simulink model "Matrix12"  (R2021a)
settings: Solver=VariableStepAuto  StartTime=0.0  StopTime=1  RelTol=1e-3
undefined symbols (not defined in the file): DiscIntNeverNeededParam
libraries: spsDiodeLib x18, spsIGBTLib x18, simulink x6, spsIGBTDiodeLib x6, spsSeriesRLCBranchLib x4, spsThreePhaseVIMeasurementLib x3, spsSaturableTransformerLib x3, spsabctoAlphaBetaZeroLib x2, spsAlphaBetaZerotoabcLib x1, pid_lib x1, spsSecondOrderFilterLib x1, spsThreePhaseSeriesRLCBranchLib x1
(part 2 of 2)

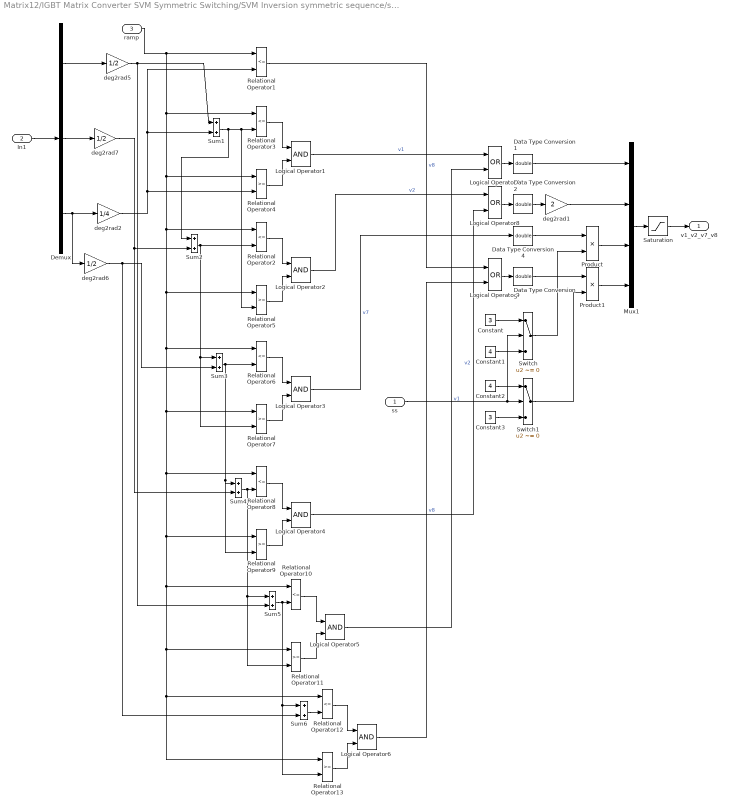
== system Matrix12/IGBT Matrix Converter SVM Symmetric Switching/SVM Inversion symmetric sequence/symmetric sequence ==
  ss : Inport
  In1 : Inport  Port=2
  ramp : Inport  Port=3
  Constant : Constant  Value=3
  Constant1 : Constant  Value=4
  Constant2 : Constant  Value=4
  Constant3 : Constant  Value=3
  Data Type Conversion{1..2,4..5} (4 alike) : DataTypeConversion  OutDataTypeStr=double
  Demux : Demux  Outputs=3
  Logical Operator{1..6} (6 alike) : Logic  AllPortsSameDT=off  OutDataTypeStr=boolean
  Logical Operator7 : Logic  Operator=OR  AllPortsSameDT=off  OutDataTypeStr=boolean
  Logical Operator8 : Logic  Operator=OR  AllPortsSameDT=off  OutDataTypeStr=boolean
  Logical Operator9 : Logic  Operator=OR  AllPortsSameDT=off  OutDataTypeStr=boolean
  Mux1 : Mux
  Product : Product  RndMeth=Zero
  Product1 : Product  RndMeth=Zero
  Relational Operator{1..3,6,8,10,12} (7 alike) : RelationalOperator  Operator=<=  RndMeth=Nearest  InputSameDT=on
  Relational Operator{4..5,7,9,11,13} (6 alike) : RelationalOperator  RndMeth=Nearest  InputSameDT=on
  Saturation : Saturate  UpperLimit=4  LowerLimit=1
  Sum{1..6} (6 alike) : Sum
  Switch : Switch  Criteria=u2 ~= 0
  Switch1 : Switch  Criteria=u2 ~= 0
  deg2rad1 : Gain  Gain=2
  deg2rad2 : Gain  Gain=1/4
  deg2rad5 : Gain  Gain=1/2
  deg2rad6 : Gain  Gain=1/2
  deg2rad7 : Gain  Gain=1/2
  v1_v2_v7_v8 : Outport  VectorParamsAs1DForOutWhenUnconnected=off
  wires:
  ss/1 -> Switch/2, Switch1/2
  Switch1/1 -> Product1/2
  Switch/1 -> Product/2
  Constant2/1 -> Switch1/1
  Constant3/1 -> Switch1/3
  Constant/1 -> Switch/1
  Constant1/1 -> Switch/3
  Product1/1 -> Mux1/4
  Product/1 -> Mux1/3
  Data Type Conversion5/1 -> Product1/1
  Data Type Conversion4/1 -> Product/1
  Data Type Conversion2/1 -> deg2rad1/1
  Data Type Conversion1/1 -> Mux1/1
  Logical Operator7/1 -> Data Type Conversion1/1
  Relational Operator1/1 -> Logical Operator9/1  "v8"
  Logical Operator1/1 -> Logical Operator7/1  "v1"
  Logical Operator6/1 -> Logical Operator9/2  "v8"
  Sum6/1 -> Relational Operator12/2
  Relational Operator13/1 -> Logical Operator6/2
  Relational Operator12/1 -> Logical Operator6/1
  Logical Operator5/1 -> Logical Operator7/2  "v1"
  Sum5/1 -> Relational Operator13/2, Sum6/1, Relational Operator10/2
  Relational Operator11/1 -> Logical Operator5/2
  Relational Operator10/1 -> Logical Operator5/1
  Logical Operator4/1 -> Logical Operator8/2  "v2"
  deg2rad7/1 -> Sum2/2, Sum4/2
  Demux/2 -> deg2rad7/1
  Sum4/1 -> Sum5/1, Relational Operator11/2, Relational Operator8/2
  Relational Operator9/1 -> Logical Operator4/2
  Relational Operator8/1 -> Logical Operator4/1
  deg2rad6/1 -> Sum6/2, Sum3/2
  Sum3/1 -> Relational Operator9/2, Sum4/1, Relational Operator6/2
  Logical Operator3/1 -> Data Type Conversion4/1  "v7"
  Relational Operator7/1 -> Logical Operator3/2
  Relational Operator6/1 -> Logical Operator3/1
  Logical Operator2/1 -> Logical Operator8/1  "v2"
  Sum2/1 -> Relational Operator7/2, Sum3/1, Relational Operator2/2
  Relational Operator5/1 -> Logical Operator2/2
  Relational Operator2/1 -> Logical Operator2/1
  deg2rad5/1 -> Sum5/2, Sum1/1
  Demux/1 -> deg2rad5/1
  deg2rad2/1 -> Sum1/2, Relational Operator1/2, Relational Operator4/2
  Sum1/1 -> Sum2/1, Relational Operator5/2, Relational Operator3/2
  Relational Operator4/1 -> Logical Operator1/2
  Relational Operator3/1 -> Logical Operator1/1
  Saturation/1 -> v1_v2_v7_v8/1
  Logical Operator9/1 -> Data Type Conversion5/1
  Logical Operator8/1 -> Data Type Conversion2/1
  deg2rad1/1 -> Mux1/2
  In1/1 -> Demux/1
  ramp/1 -> Relational Operator1/1, Relational Operator13/1, Relational Operator12/1, Relational Operator11/1, Relational Operator10/1, Relational Operator9/1, Relational Operator8/1, Relational Operator7/1, Relational Operator6/1, Relational Operator5/1, Relational Operator2/1, Relational Operator4/1, Relational Operator3/1
  Mux1/1 -> Saturation/1
  Demux/3 -> deg2rad6/1, deg2rad2/1

== system Matrix12/IGBT Matrix Converter SVM Symmetric Switching/SVM Rectification symmetric sequence/Calculate duty-cycles ==
  deg_mag : Inport
  Trigger : TriggerPort  VariantControl=Variant
  Constant : Constant  Value=pi/3
  Constant1 : Constant
  Demux : Demux  Outputs=2
  Mux : Mux  Inputs=2
  Mux1 : Mux  Inputs=2
  Product : Product  Inputs=**  RndMeth=Zero
  Sum : Sum  Inputs=+-
  Sum of Elements : Sum  Inputs=+
  Sum1 : Sum  Inputs=-+
  Sum2 : Sum  Inputs=-+
  Trigonometric Function : Trigonometry  Operator=cos
  Trigonometric Function1 : Trigonometry
  deg2rad : Gain  Gain=pi/180
  deg2rad1 : Gain  Gain=0.5/0.866
  d1_d2_d0 : Outport  VectorParamsAs1DForOutWhenUnconnected=off
  wires:
  Sum of Elements/1 -> Sum2/1
  Constant1/1 -> Sum2/2
  Sum2/1 -> Mux1/2  "d0"
  Mux1/1 -> d1_d2_d0/1
  Product/1 -> Sum of Elements/1, Mux1/1  "d1 d2"
  Constant/1 -> Sum1/2
  Mux/1 -> Trigonometric Function1/1, Trigonometric Function/1
  Sum1/1 -> Mux/2
  deg2rad/1 -> Sum1/1, Mux/1  "theta"
  Sum/1 -> Product/1
  deg2rad1/1 -> Sum/2
  Trigonometric Function1/1 -> deg2rad1/1
  Trigonometric Function/1 -> Sum/1
  Demux/2 -> Product/2  "mag"
  Demux/1 -> deg2rad/1
  deg_mag/1 -> Demux/1

== system Matrix12/IGBT Matrix Converter SVM Symmetric Switching/SVM Rectification symmetric sequence/Triggered Subsystem ==
  In1 : Inport
  Trigger : TriggerPort  VariantControl=Variant
  Out1 : Outport  VectorParamsAs1DForOutWhenUnconnected=off
  wires:
  In1/1 -> Out1/1

== system Matrix12/IGBT Matrix Converter SVM Symmetric Switching/SVM Rectification symmetric sequence/abc 2 alpha-beta ==
  Vabc : Inport
  Demux : Demux  Outputs=3
      settings: DisplayOption=none
  Gain : Gain  Gain=1/2  SaturateOnIntegerOverflow=on  OutDataTypeStr=Inherit: Same as input  ParamDataTypeStr=Inherit: Same as input
  Gain1 : Gain  Gain=1/2  SaturateOnIntegerOverflow=on  OutDataTypeStr=Inherit: Same as input  ParamDataTypeStr=Inherit: Same as input
  Gain2 : Gain  Gain=sqrt(2/3)  SaturateOnIntegerOverflow=on  OutDataTypeStr=Inherit: Same as input  ParamDataTypeStr=Inherit: Same as input
  Gain3 : Gain  Gain=sqrt(3)/2  SaturateOnIntegerOverflow=on  OutDataTypeStr=Inherit: Same as input  ParamDataTypeStr=Inherit: Same as input
  Gain4 : Gain  Gain=sqrt(3)/2  SaturateOnIntegerOverflow=on  OutDataTypeStr=Inherit: Same as input  ParamDataTypeStr=Inherit: Same as input
  Gain5 : Gain  Gain=sqrt(2/3)  SaturateOnIntegerOverflow=on  OutDataTypeStr=Inherit: Same as input  ParamDataTypeStr=Inherit: Same as input
  Sum : Sum  Inputs=+--  InputSameDT=on  SaturateOnIntegerOverflow=on  OutDataTypeStr=Inherit: Same as first input
  Sum1 : Sum  Inputs=+-  InputSameDT=on  SaturateOnIntegerOverflow=on  OutDataTypeStr=Inherit: Same as first input
  Valpha : Outport  VectorParamsAs1DForOutWhenUnconnected=off
  Vbeta : Outport  Port=2  VectorParamsAs1DForOutWhenUnconnected=off
  wires:
  Gain5/1 -> Vbeta/1
  Gain2/1 -> Valpha/1
  Vabc/1 -> Demux/1
  Gain3/1 -> Sum1/1
  Gain4/1 -> Sum1/2
  Sum1/1 -> Gain5/1
  Sum/1 -> Gain2/1
  Gain1/1 -> Sum/3
  Gain/1 -> Sum/2
  Demux/1 -> Sum/1
  Demux/2 -> Gain/1, Gain3/1
  Demux/3 -> Gain1/1, Gain4/1

== system Matrix12/IGBT Matrix Converter SVM Symmetric Switching/SVM Rectification symmetric sequence/alpha-beta 2 deg-mag ==
  Valpha : Inport
  Vbeta : Inport  Port=2
  Constant1 : Constant  Value=180
  Constant2 : Constant  Value=-360
  Constant20 : Constant  Value=30
  Math Function : Math  Operator=square  SignedPower=on  SaturateOnIntegerOverflow=on
  Math Function1 : Math  Operator=sqrt  SignedPower=on  SaturateOnIntegerOverflow=on
  Mux1 : Mux  Inputs=2
  Relational Operator2 : RelationalOperator  Operator=>  RndMeth=Nearest  InputSameDT=on
  Sum of Elements : Sum  Inputs=+
  Sum1 : Sum  Inputs=|++
  Sum2 : Sum  Inputs=|++
  Switch : Switch  Criteria=u2 ~= 0
  Trigonometric Function : Trigonometry  Operator=atan2
  rad2deg : Gain  Gain=180/pi  SaturateOnIntegerOverflow=on  OutDataTypeStr=Inherit: Same as input  ParamDataTypeStr=Inherit: Same as input
  Vdeg : Outport  VectorParamsAs1DForOutWhenUnconnected=off
  Vmag : Outport  Port=2  VectorParamsAs1DForOutWhenUnconnected=off
  wires:
  Trigonometric Function/1 -> rad2deg/1
  Valpha/1 -> Trigonometric Function/2, Mux1/1
  Mux1/1 -> Math Function/1
  Math Function/1 -> Sum of Elements/1
  Sum of Elements/1 -> Math Function1/1
  Vbeta/1 -> Trigonometric Function/1, Mux1/2
  Math Function1/1 -> Vmag/1
  rad2deg/1 -> Sum1/1
  Constant20/1 -> Sum1/2
  Sum1/1 -> Relational Operator2/1, Switch/3, Sum2/1
  Relational Operator2/1 -> Switch/2
  Switch/1 -> Vdeg/1
  Constant1/1 -> Relational Operator2/2
  Sum2/1 -> Switch/1
  Constant2/1 -> Sum2/2

== system Matrix12/IGBT Matrix Converter SVM Symmetric Switching/SVM Rectification symmetric sequence/choose zero-vector ==
  sector : Inport
  Compare To Constant : simulink/Logic and Bit Operations/Compare To Constant  relop===  const=1  OutDataTypeStr=uint8  ZeroCross=off
  Compare To Constant1 : simulink/Logic and Bit Operations/Compare To Constant  relop===  const=4  OutDataTypeStr=uint8  ZeroCross=off
  Compare To Constant2 : simulink/Logic and Bit Operations/Compare To Constant  relop===  const=2  OutDataTypeStr=uint8  ZeroCross=off
  Compare To Constant3 : simulink/Logic and Bit Operations/Compare To Constant  relop===  const=5  OutDataTypeStr=uint8  ZeroCross=off
  Compare To Constant4 : simulink/Logic and Bit Operations/Compare To Constant  relop===  const=3  OutDataTypeStr=uint8  ZeroCross=off
  Compare To Constant5 : simulink/Logic and Bit Operations/Compare To Constant  relop===  const=6  OutDataTypeStr=uint8  ZeroCross=off
  Data Type Conversion1 : DataTypeConversion  OutDataTypeStr=double
  Data Type Conversion2 : DataTypeConversion  OutDataTypeStr=double
  Data Type Conversion3 : DataTypeConversion  OutDataTypeStr=double
  Logical Operator1 : Logic  Operator=OR  AllPortsSameDT=off  OutDataTypeStr=boolean
  Logical Operator2 : Logic  Operator=OR  AllPortsSameDT=off  OutDataTypeStr=boolean
  Logical Operator8 : Logic  Operator=OR  AllPortsSameDT=off  OutDataTypeStr=boolean
  MinMax1 : MinMax  Function=max
  Mux1 : Mux  Inputs=3
  Saturation1 : Saturate  UpperLimit=3  LowerLimit=1
  deg2rad2 : Gain  Gain=2
  deg2rad4 : Gain  Gain=3
  zv : Outport  VectorParamsAs1DForOutWhenUnconnected=off
  wires:
  Compare To Constant/1 -> Logical Operator8/1
  Compare To Constant1/1 -> Logical Operator8/2
  Compare To Constant2/1 -> Logical Operator1/1
  Compare To Constant3/1 -> Logical Operator1/2
  Compare To Constant4/1 -> Logical Operator2/1
  Compare To Constant5/1 -> Logical Operator2/2
  Logical Operator8/1 -> Data Type Conversion1/1
  Logical Operator1/1 -> Data Type Conversion2/1
  Logical Operator2/1 -> Data Type Conversion3/1
  Data Type Conversion1/1 -> Mux1/1
  Data Type Conversion2/1 -> deg2rad2/1
  Data Type Conversion3/1 -> deg2rad4/1
  Mux1/1 -> Saturation1/1
  deg2rad4/1 -> Mux1/3
  deg2rad2/1 -> Mux1/2
  Saturation1/1 -> MinMax1/1
  MinMax1/1 -> zv/1
  sector/1 -> Compare To Constant/1, Compare To Constant1/1, Compare To Constant2/1, Compare To Constant3/1, Compare To Constant4/1, Compare To Constant5/1

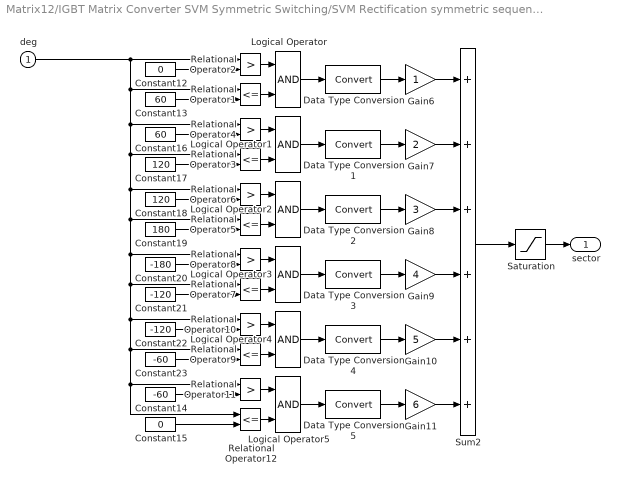
== system Matrix12/IGBT Matrix Converter SVM Symmetric Switching/SVM Rectification symmetric sequence/sector ==
  deg : Inport
  Constant12 : Constant  Value=0
  Constant13 : Constant  Value=60
  Constant14 : Constant  Value=-60
  Constant15 : Constant  Value=0
  Constant16 : Constant  Value=60
  Constant17 : Constant  Value=120
  Constant18 : Constant  Value=120
  Constant19 : Constant  Value=180
  Constant20 : Constant  Value=-180
  Constant21 : Constant  Value=-120
  Constant22 : Constant  Value=-120
  Constant23 : Constant  Value=-60
  Data Type Conversion{,1..5} (6 alike) : DataTypeConversion  SaturateOnIntegerOverflow=on  RndMeth=Zero
  Gain10 : Gain  Gain=5  SaturateOnIntegerOverflow=on  OutDataTypeStr=Inherit: Same as input  ParamDataTypeStr=Inherit: Same as input
  Gain11 : Gain  Gain=6  SaturateOnIntegerOverflow=on  OutDataTypeStr=Inherit: Same as input  ParamDataTypeStr=Inherit: Same as input
  Gain6 : Gain  SaturateOnIntegerOverflow=on  OutDataTypeStr=Inherit: Same as input  ParamDataTypeStr=Inherit: Same as input
  Gain7 : Gain  Gain=2  SaturateOnIntegerOverflow=on  OutDataTypeStr=Inherit: Same as input  ParamDataTypeStr=Inherit: Same as input
  Gain8 : Gain  Gain=3  SaturateOnIntegerOverflow=on  OutDataTypeStr=Inherit: Same as input  ParamDataTypeStr=Inherit: Same as input
  Gain9 : Gain  Gain=4  SaturateOnIntegerOverflow=on  OutDataTypeStr=Inherit: Same as input  ParamDataTypeStr=Inherit: Same as input
  Logical Operator{,1..5} (6 alike) : Logic
  Relational Operator{1,3,5,7,9,12} (6 alike) : RelationalOperator  Operator=<=  RndMeth=Nearest  InputSameDT=on
  Relational Operator{2,4,6,8,10..11} (6 alike) : RelationalOperator  Operator=>  RndMeth=Nearest  InputSameDT=on
  Saturation : Saturate  UpperLimit=6  LowerLimit=1
  Sum2 : Sum  Inputs=++++++  InputSameDT=on  SaturateOnIntegerOverflow=on  OutDataTypeStr=Inherit: Same as first input
  sector : Outport  VectorParamsAs1DForOutWhenUnconnected=off
  wires:
  deg/1 -> Relational Operator2/1, Relational Operator1/1, Relational Operator4/1, Relational Operator3/1, Relational Operator6/1, Relational Operator5/1, Relational Operator8/1, Relational Operator7/1, Relational Operator10/1, Relational Operator9/1, Relational Operator11/1, Relational Operator12/1
  Saturation/1 -> sector/1
  Data Type Conversion5/1 -> Gain11/1
  Data Type Conversion4/1 -> Gain10/1
  Data Type Conversion3/1 -> Gain9/1
  Data Type Conversion2/1 -> Gain8/1
  Data Type Conversion1/1 -> Gain7/1
  Data Type Conversion/1 -> Gain6/1
  Relational Operator2/1 -> Logical Operator/1
  Relational Operator1/1 -> Logical Operator/2
  Logical Operator/1 -> Data Type Conversion/1
  Constant12/1 -> Relational Operator2/2
  Constant13/1 -> Relational Operator1/2
  Relational Operator4/1 -> Logical Operator1/1
  Relational Operator3/1 -> Logical Operator1/2
  Logical Operator1/1 -> Data Type Conversion1/1
  Constant16/1 -> Relational Operator4/2
  Constant17/1 -> Relational Operator3/2
  Relational Operator6/1 -> Logical Operator2/1
  Relational Operator5/1 -> Logical Operator2/2
  Logical Operator2/1 -> Data Type Conversion2/1
  Constant18/1 -> Relational Operator6/2
  Constant19/1 -> Relational Operator5/2
  Relational Operator8/1 -> Logical Operator3/1
  Relational Operator7/1 -> Logical Operator3/2
  Logical Operator3/1 -> Data Type Conversion3/1
  Constant20/1 -> Relational Operator8/2
  Constant21/1 -> Relational Operator7/2
  Relational Operator10/1 -> Logical Operator4/1
  Relational Operator9/1 -> Logical Operator4/2
  Logical Operator4/1 -> Data Type Conversion4/1
  Constant22/1 -> Relational Operator10/2
  Constant23/1 -> Relational Operator9/2
  Relational Operator11/1 -> Logical Operator5/1
  Relational Operator12/1 -> Logical Operator5/2
  Logical Operator5/1 -> Data Type Conversion5/1
  Constant14/1 -> Relational Operator11/2
  Constant15/1 -> Relational Operator12/2
  Gain6/1 -> Sum2/1
  Gain7/1 -> Sum2/2
  Gain8/1 -> Sum2/3
  Gain9/1 -> Sum2/4
  Gain10/1 -> Sum2/5
  Gain11/1 -> Sum2/6
  Sum2/1 -> Saturation/1

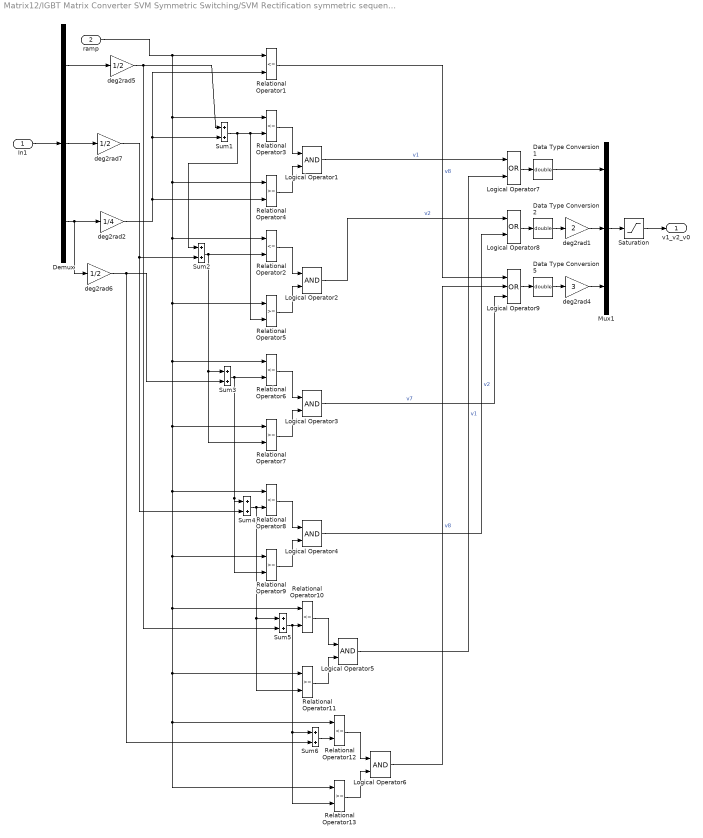
== system Matrix12/IGBT Matrix Converter SVM Symmetric Switching/SVM Rectification symmetric sequence/symmetric sequence ==
  In1 : Inport
  ramp : Inport  Port=2
  Data Type Conversion1 : DataTypeConversion  OutDataTypeStr=double
  Data Type Conversion2 : DataTypeConversion  OutDataTypeStr=double
  Data Type Conversion5 : DataTypeConversion  OutDataTypeStr=double
  Demux : Demux  Outputs=3
  Logical Operator{1..6} (6 alike) : Logic  AllPortsSameDT=off  OutDataTypeStr=boolean
  Logical Operator7 : Logic  Operator=OR  AllPortsSameDT=off  OutDataTypeStr=boolean
  Logical Operator8 : Logic  Operator=OR  AllPortsSameDT=off  OutDataTypeStr=boolean
  Logical Operator9 : Logic  Operator=OR  Inputs=3  AllPortsSameDT=off  OutDataTypeStr=boolean
  Mux1 : Mux  Inputs=3
  Relational Operator{1..3,6,8,10,12} (7 alike) : RelationalOperator  Operator=<=  RndMeth=Nearest  InputSameDT=on
  Relational Operator{4..5,7,9,11,13} (6 alike) : RelationalOperator  RndMeth=Nearest  InputSameDT=on
  Saturation : Saturate  UpperLimit=3  LowerLimit=1
  Sum{1..6} (6 alike) : Sum
  deg2rad1 : Gain  Gain=2
  deg2rad2 : Gain  Gain=1/4
  deg2rad4 : Gain  Gain=3
  deg2rad5 : Gain  Gain=1/2
  deg2rad6 : Gain  Gain=1/2
  deg2rad7 : Gain  Gain=1/2
  v1_v2_v0 : Outport  VectorParamsAs1DForOutWhenUnconnected=off
  wires:
  Demux/3 -> deg2rad2/1, deg2rad6/1
  Mux1/1 -> Saturation/1
  ramp/1 -> Relational Operator3/1, Relational Operator4/1, Relational Operator2/1, Relational Operator5/1, Relational Operator6/1, Relational Operator7/1, Relational Operator8/1, Relational Operator9/1, Relational Operator10/1, Relational Operator11/1, Relational Operator12/1, Relational Operator13/1, Relational Operator1/1
  In1/1 -> Demux/1
  deg2rad1/1 -> Mux1/2
  deg2rad4/1 -> Mux1/3
  Logical Operator8/1 -> Data Type Conversion2/1
  Logical Operator9/1 -> Data Type Conversion5/1
  Saturation/1 -> v1_v2_v0/1
  Relational Operator3/1 -> Logical Operator1/1
  Relational Operator4/1 -> Logical Operator1/2
  Sum1/1 -> Relational Operator3/2, Relational Operator5/2, Sum2/1
  deg2rad2/1 -> Relational Operator4/2, Relational Operator1/2, Sum1/2
  Demux/1 -> deg2rad5/1
  deg2rad5/1 -> Sum1/1, Sum5/2
  Relational Operator2/1 -> Logical Operator2/1
  Relational Operator5/1 -> Logical Operator2/2
  Sum2/1 -> Relational Operator2/2, Sum3/1, Relational Operator7/2
  Logical Operator2/1 -> Logical Operator8/1  "v2"
  Relational Operator6/1 -> Logical Operator3/1
  Relational Operator7/1 -> Logical Operator3/2
  Sum3/1 -> Relational Operator6/2, Sum4/1, Relational Operator9/2
  deg2rad6/1 -> Sum3/2, Sum6/2
  Relational Operator8/1 -> Logical Operator4/1
  Relational Operator9/1 -> Logical Operator4/2
  Sum4/1 -> Relational Operator8/2, Relational Operator11/2, Sum5/1
  Demux/2 -> deg2rad7/1
  deg2rad7/1 -> Sum4/2, Sum2/2
  Logical Operator4/1 -> Logical Operator8/2  "v2"
  Relational Operator10/1 -> Logical Operator5/1
  Relational Operator11/1 -> Logical Operator5/2
  Sum5/1 -> Relational Operator10/2, Sum6/1, Relational Operator13/2
  Logical Operator5/1 -> Logical Operator7/2  "v1"
  Relational Operator12/1 -> Logical Operator6/1
  Relational Operator13/1 -> Logical Operator6/2
  Sum6/1 -> Relational Operator12/2
  Logical Operator6/1 -> Logical Operator9/2  "v8"
  Logical Operator1/1 -> Logical Operator7/1  "v1"
  Relational Operator1/1 -> Logical Operator9/1  "v8"
  Logical Operator7/1 -> Data Type Conversion1/1
  Data Type Conversion1/1 -> Mux1/1
  Data Type Conversion2/1 -> deg2rad1/1
  Data Type Conversion5/1 -> deg2rad4/1
  Logical Operator3/1 -> Logical Operator9/3  "v7"

== system Matrix12/IGBT Matrix Converter SVM Symmetric Switching/matrix converter switching/Subsystem1 ==
  In1 : Inport
  In2 : Inport  Port=2
  In3 : Inport  Port=3
  In4 : Inport  Port=4
  Data Type Conversion : DataTypeConversion  OutDataTypeStr=double
  Logical Operator : Logic  AllPortsSameDT=off  OutDataTypeStr=boolean
  Logical Operator1 : Logic  AllPortsSameDT=off  OutDataTypeStr=boolean
  Logical Operator2 : Logic  Operator=OR  AllPortsSameDT=off  OutDataTypeStr=boolean
  Out1 : Outport  VectorParamsAs1DForOutWhenUnconnected=off
  wires:
  In4/1 -> Logical Operator1/2
  In3/1 -> Logical Operator1/1
  Logical Operator2/1 -> Data Type Conversion/1
  In2/1 -> Logical Operator/2
  In1/1 -> Logical Operator/1
  Logical Operator1/1 -> Logical Operator2/2
  Logical Operator/1 -> Logical Operator2/1
  Data Type Conversion/1 -> Out1/1

== system Matrix12/IGBT Matrix Converter SVM Symmetric Switching/matrix converter switching/Subsystem2 ==
  In1 : Inport
  In2 : Inport  Port=2
  In3 : Inport  Port=3
  In4 : Inport  Port=4
  Data Type Conversion : DataTypeConversion  OutDataTypeStr=double
  Logical Operator : Logic  AllPortsSameDT=off  OutDataTypeStr=boolean
  Logical Operator1 : Logic  AllPortsSameDT=off  OutDataTypeStr=boolean
  Logical Operator2 : Logic  Operator=OR  AllPortsSameDT=off  OutDataTypeStr=boolean
  Out1 : Outport  VectorParamsAs1DForOutWhenUnconnected=off
  wires:
  In4/1 -> Logical Operator1/2
  In3/1 -> Logical Operator1/1
  Logical Operator2/1 -> Data Type Conversion/1
  In2/1 -> Logical Operator/2
  In1/1 -> Logical Operator/1
  Logical Operator1/1 -> Logical Operator2/2
  Logical Operator/1 -> Logical Operator2/1
  Data Type Conversion/1 -> Out1/1

== system Matrix12/IGBT Matrix Converter SVM Symmetric Switching/matrix converter switching/Subsystem3 ==
  In1 : Inport
  In2 : Inport  Port=2
  In3 : Inport  Port=3
  In4 : Inport  Port=4
  Data Type Conversion : DataTypeConversion  OutDataTypeStr=double
  Logical Operator : Logic  AllPortsSameDT=off  OutDataTypeStr=boolean
  Logical Operator1 : Logic  AllPortsSameDT=off  OutDataTypeStr=boolean
  Logical Operator2 : Logic  Operator=OR  AllPortsSameDT=off  OutDataTypeStr=boolean
  Out1 : Outport  VectorParamsAs1DForOutWhenUnconnected=off
  wires:
  In4/1 -> Logical Operator1/2
  In3/1 -> Logical Operator1/1
  Logical Operator2/1 -> Data Type Conversion/1
  In2/1 -> Logical Operator/2
  In1/1 -> Logical Operator/1
  Logical Operator1/1 -> Logical Operator2/2
  Logical Operator/1 -> Logical Operator2/1
  Data Type Conversion/1 -> Out1/1

== system Matrix12/IGBT Matrix Converter SVM Symmetric Switching/matrix converter switching/Subsystem4 ==
  In1 : Inport
  In2 : Inport  Port=2
  In3 : Inport  Port=3
  In4 : Inport  Port=4
  Data Type Conversion : DataTypeConversion  OutDataTypeStr=double
  Logical Operator : Logic  AllPortsSameDT=off  OutDataTypeStr=boolean
  Logical Operator1 : Logic  AllPortsSameDT=off  OutDataTypeStr=boolean
  Logical Operator2 : Logic  Operator=OR  AllPortsSameDT=off  OutDataTypeStr=boolean
  Out1 : Outport  VectorParamsAs1DForOutWhenUnconnected=off
  wires:
  In4/1 -> Logical Operator1/2
  In3/1 -> Logical Operator1/1
  Logical Operator2/1 -> Data Type Conversion/1
  In2/1 -> Logical Operator/2
  In1/1 -> Logical Operator/1
  Logical Operator1/1 -> Logical Operator2/2
  Logical Operator/1 -> Logical Operator2/1
  Data Type Conversion/1 -> Out1/1

== system Matrix12/IGBT Matrix Converter SVM Symmetric Switching/matrix converter switching/Subsystem5 ==
  In1 : Inport
  In2 : Inport  Port=2
  In3 : Inport  Port=3
  In4 : Inport  Port=4
  Data Type Conversion : DataTypeConversion  OutDataTypeStr=double
  Logical Operator : Logic  AllPortsSameDT=off  OutDataTypeStr=boolean
  Logical Operator1 : Logic  AllPortsSameDT=off  OutDataTypeStr=boolean
  Logical Operator2 : Logic  Operator=OR  AllPortsSameDT=off  OutDataTypeStr=boolean
  Out1 : Outport  VectorParamsAs1DForOutWhenUnconnected=off
  wires:
  In4/1 -> Logical Operator1/2
  In3/1 -> Logical Operator1/1
  Logical Operator2/1 -> Data Type Conversion/1
  In2/1 -> Logical Operator/2
  In1/1 -> Logical Operator/1
  Logical Operator1/1 -> Logical Operator2/2
  Logical Operator/1 -> Logical Operator2/1
  Data Type Conversion/1 -> Out1/1

== system Matrix12/IGBT Matrix Converter SVM Symmetric Switching/matrix converter switching/Subsystem6 ==
  In1 : Inport
  In2 : Inport  Port=2
  In3 : Inport  Port=3
  In4 : Inport  Port=4
  Data Type Conversion : DataTypeConversion  OutDataTypeStr=double
  Logical Operator : Logic  AllPortsSameDT=off  OutDataTypeStr=boolean
  Logical Operator1 : Logic  AllPortsSameDT=off  OutDataTypeStr=boolean
  Logical Operator2 : Logic  Operator=OR  AllPortsSameDT=off  OutDataTypeStr=boolean
  Out1 : Outport  VectorParamsAs1DForOutWhenUnconnected=off
  wires:
  In4/1 -> Logical Operator1/2
  In3/1 -> Logical Operator1/1
  Logical Operator2/1 -> Data Type Conversion/1
  In2/1 -> Logical Operator/2
  In1/1 -> Logical Operator/1
  Logical Operator1/1 -> Logical Operator2/2
  Logical Operator/1 -> Logical Operator2/1
  Data Type Conversion/1 -> Out1/1

== system Matrix12/IGBT Matrix Converter SVM Symmetric Switching/matrix converter switching/Subsystem7 ==
  In1 : Inport
  In2 : Inport  Port=2
  In3 : Inport  Port=3
  In4 : Inport  Port=4
  Data Type Conversion : DataTypeConversion  OutDataTypeStr=double
  Logical Operator : Logic  AllPortsSameDT=off  OutDataTypeStr=boolean
  Logical Operator1 : Logic  AllPortsSameDT=off  OutDataTypeStr=boolean
  Logical Operator2 : Logic  Operator=OR  AllPortsSameDT=off  OutDataTypeStr=boolean
  Out1 : Outport  VectorParamsAs1DForOutWhenUnconnected=off
  wires:
  In4/1 -> Logical Operator1/2
  In3/1 -> Logical Operator1/1
  Logical Operator2/1 -> Data Type Conversion/1
  In2/1 -> Logical Operator/2
  In1/1 -> Logical Operator/1
  Logical Operator1/1 -> Logical Operator2/2
  Logical Operator/1 -> Logical Operator2/1
  Data Type Conversion/1 -> Out1/1

== system Matrix12/IGBT Matrix Converter SVM Symmetric Switching/matrix converter switching/Subsystem8 ==
  In1 : Inport
  In2 : Inport  Port=2
  In3 : Inport  Port=3
  In4 : Inport  Port=4
  Data Type Conversion : DataTypeConversion  OutDataTypeStr=double
  Logical Operator : Logic  AllPortsSameDT=off  OutDataTypeStr=boolean
  Logical Operator1 : Logic  AllPortsSameDT=off  OutDataTypeStr=boolean
  Logical Operator2 : Logic  Operator=OR  AllPortsSameDT=off  OutDataTypeStr=boolean
  Out1 : Outport  VectorParamsAs1DForOutWhenUnconnected=off
  wires:
  In4/1 -> Logical Operator1/2
  In3/1 -> Logical Operator1/1
  Logical Operator2/1 -> Data Type Conversion/1
  In2/1 -> Logical Operator/2
  In1/1 -> Logical Operator/1
  Logical Operator1/1 -> Logical Operator2/2
  Logical Operator/1 -> Logical Operator2/1
  Data Type Conversion/1 -> Out1/1

== system Matrix12/IGBT Matrix Converter SVM Symmetric Switching/matrix converter switching/Subsystem9 ==
  In1 : Inport
  In2 : Inport  Port=2
  In3 : Inport  Port=3
  In4 : Inport  Port=4
  Data Type Conversion : DataTypeConversion  OutDataTypeStr=double
  Logical Operator : Logic  AllPortsSameDT=off  OutDataTypeStr=boolean
  Logical Operator1 : Logic  AllPortsSameDT=off  OutDataTypeStr=boolean
  Logical Operator2 : Logic  Operator=OR  AllPortsSameDT=off  OutDataTypeStr=boolean
  Out1 : Outport  VectorParamsAs1DForOutWhenUnconnected=off
  wires:
  In4/1 -> Logical Operator1/2
  In3/1 -> Logical Operator1/1
  Logical Operator2/1 -> Data Type Conversion/1
  In2/1 -> Logical Operator/2
  In1/1 -> Logical Operator/1
  Logical Operator1/1 -> Logical Operator2/2
  Logical Operator/1 -> Logical Operator2/1
  Data Type Conversion/1 -> Out1/1
